simulink model "inv_pen_IC_compare_mar2016"  (R2015b)
settings: Solver=ode45  StartTime=0.0  StopTime=16  MaxStep=0.001  RelTol=1e-3
values from neighbouring files (symbols this model uses):
  g = 9.81    [inverted_pendulum_Feb28_2016.m]
  K1 = K(1)    [inverted_pendulum_Feb28_2016.m]
  K2 = K(2)    [inverted_pendulum_Feb28_2016.m]
  K3 = K(3)    [inverted_pendulum_Feb28_2016.m]
  K4 = K(4)    [inverted_pendulum_Feb28_2016.m]
  l = 0.5    [inverted_pendulum_Feb28_2016.m]
  M = 2    [inverted_pendulum_Feb28_2016.m]
  m = .1    (= 0.1)    [inverted_pendulum_Feb28_2016.m]
libraries: simulink x1
settings Model: Creator=Thomas Chmielewski  LastModifiedBy=DR_C
settings DataIOCC: SaveFormat=Array  SignalLoggingSaveFormat=ModelDataLogs
settings OptimizationCC: ExpressionDepthLimit=2147483647  InitFltsAndDblsToZero=on
settings DebuggingCC: SaveWithParameterizedLinksMsg=none  UnderspecifiedInitializationDetection=Classic  MergeDetectMultiDrivingBlocksExec=none  SolverPrmCheckMsg=warning  FcnCallInpInsideContextMsg=UseLocalSettings  StateNameClashWarn=warning
settings HardwareCC: ProdBitPerPointer=32  ProdLargestAtomicFloat=None  ProdIntDivRoundTo=Undefined  ProdEndianess=Unspecified  ProdWordSize=32  ProdHWDeviceType=32-bit Generic
settings GRTTargetCC: TargetFcnLib=ansi_tfl_tmw.mat  GeneratePreprocessorConditionals=Disable all  CombineOutputUpdateFcns=off  GRTInterface=on
settings ConfigComp: CovModelRefEnable=Off  CovSFcnEnable=off

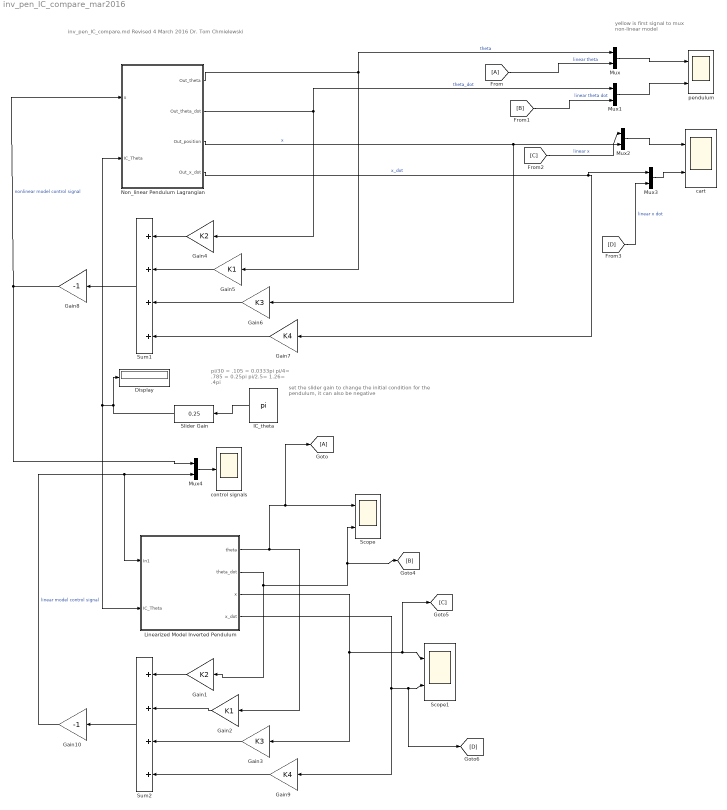
== system inv_pen_IC_compare_mar2016 ==
  note: set the slider gain to change the initial condition
      | for the pendulum, it can also be negative
  note: inv_pen_IC_compare.md
      | Revised 4 March 2016
      | Dr. Tom Chmielewski
  note: yellow is first signal to mux
      | non-linear model
  note: pi/30 = .105 = 0.0333pi
      | pi/4= .785 = 0.25pi
      | pi/2.5= 1.26= .4pi
  " cart" : Scope  NumInputPorts=2
  " control signals" : Scope
  " pendulum" : Scope  NumInputPorts=2
  Display : Display
  Gain1 : Gain  Gain=K2
  Gain10 : Gain  Gain=-1
  Gain2 : Gain  Gain=K1
  Gain3 : Gain  Gain=K3
  Gain4 : Gain  Gain=K2
  Gain5 : Gain  Gain=K1
  Gain6 : Gain  Gain=K3
  Gain7 : Gain  Gain=K4
  Gain8 : Gain  Gain=-1
  Gain9 : Gain  Gain=K4
  IC_theta : Constant  Value=pi
  Linearized Model Inverted Pendulum : Subsystem
  Mux{,1..4} (5 alike) : Mux  Inputs=2
  Non_linear Pendulum Lagrangian : Subsystem
  Scope : Scope  NumInputPorts=2
  Scope1 : Scope  NumInputPorts=2
  Slider Gain : simulink/Math Operations/Slider Gain  low=-0.4  gain=0.25  high=0.4
  Sum1 : Sum  Inputs=++++
  Sum2 : Sum  Inputs=++++
  wires:
  Gain4/1 -> Sum1/1
  Gain5/1 -> Sum1/2
  Gain6/1 -> Sum1/3
  Gain7/1 -> Sum1/4
  Sum1/1 -> Gain8/1
  Non_linear Pendulum Lagrangian/3(Out_position) -> Gain6/1, Mux2/1  "x"
  Gain8/1 -> Mux4/1, Non_linear Pendulum Lagrangian/1(u)  "nonlinear model control signal"
  Non_linear Pendulum Lagrangian/4(Out_x_dot) -> Gain7/1, Mux3/1  "x_dot"
  Non_linear Pendulum Lagrangian/1(Out_theta) -> Mux/1, Gain5/1  "theta"
  Non_linear Pendulum Lagrangian/2(Out_theta_dot) -> Gain4/1, Mux1/1  "theta_dot"
  Gain1/1 -> Sum2/1
  Gain2/1 -> Sum2/2
  Gain3/1 -> Sum2/3
  Gain9/1 -> Sum2/4
  Sum2/1 -> Gain10/1
  Linearized Model Inverted Pendulum/1(theta) -> Gain2/1, Scope/1, [A]
  Linearized Model Inverted Pendulum/2(theta_dot) -> Gain1/1, Scope/2, [B]
  Linearized Model Inverted Pendulum/3(x) -> Gain3/1, Scope1/1, [C]
  Linearized Model Inverted Pendulum/4(x_dot) -> Gain9/1, Scope1/2, [D]
  Mux/1 -> " pendulum"/1
  Mux1/1 -> " pendulum"/2
  Mux2/1 -> " cart"/1
  Mux3/1 -> " cart"/2
  [B] -> Mux1/2  "linear theta dot"
  [C] -> Mux2/2  "linear x"
  [D] -> Mux3/2  "linear x dot"
  [A] -> Mux/2  "linear theta"
  Gain10/1 -> Linearized Model Inverted Pendulum/1(In1), Mux4/2  "linear model control signal"
  Slider Gain/1 -> Non_linear Pendulum Lagrangian/2(IC_Theta), Linearized Model Inverted Pendulum/2(IC_Theta), Display/1
  IC_theta/1 -> Slider Gain/1
  Mux4/1 -> " control signals"/1

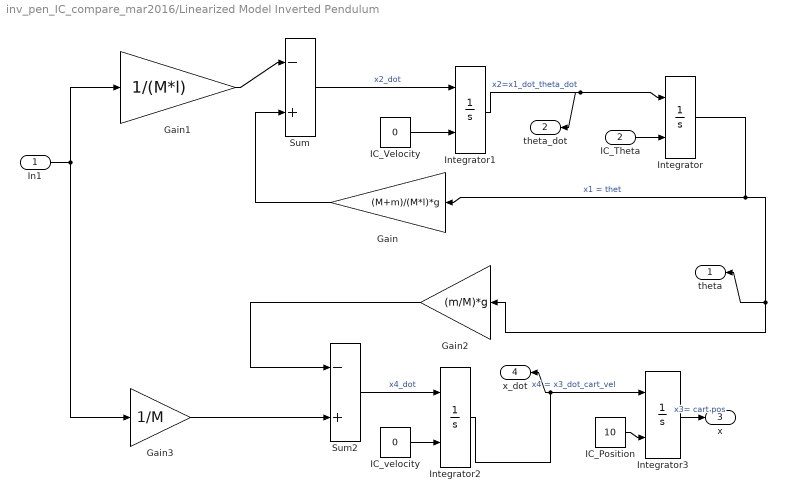
== system inv_pen_IC_compare_mar2016/Linearized Model Inverted Pendulum ==
  In1 : Inport
  IC_Theta : Inport  Port=2
  Gain : Gain  Gain=(M+m)/(M*l)*g
  Gain1 : Gain  Gain=1/(M*l)
  Gain2 : Gain  Gain=(m/M)*g
  Gain3 : Gain  Gain=1/M
  IC_Position : Constant  Value=10
  IC_Velocity : Constant  Value=0
  IC_velocity : Constant  Value=0
  Integrator{,1..3} (4 alike) : Integrator  InitialConditionSource=external
  Sum : Sum  Inputs=|-+
  Sum2 : Sum  Inputs=-+
  theta : Outport
  theta_dot : Outport  Port=2
  x : Outport  Port=3
  x_dot : Outport  Port=4
  wires:
  Integrator/1 -> Gain/1, Gain2/1, theta/1  "x1 = thet"
  Integrator1/1 -> Integrator/1, theta_dot/1  "x2=x1_dot_theta_dot"
  Sum/1 -> Integrator1/1  "x2_dot"
  Gain/1 -> Sum/2
  Gain1/1 -> Sum/1
  Integrator2/1 -> Integrator3/1, x_dot/1  "x4 = x3_dot_cart_vel"
  Sum2/1 -> Integrator2/1  "x4_dot"
  Gain2/1 -> Sum2/1
  Gain3/1 -> Sum2/2
  IC_Theta/1 -> Integrator/2
  In1/1 -> Gain3/1, Gain1/1
  IC_velocity/1 -> Integrator2/2
  IC_Position/1 -> Integrator3/2
  IC_Velocity/1 -> Integrator1/2
  Integrator3/1 -> x/1  "x3= cart pos"

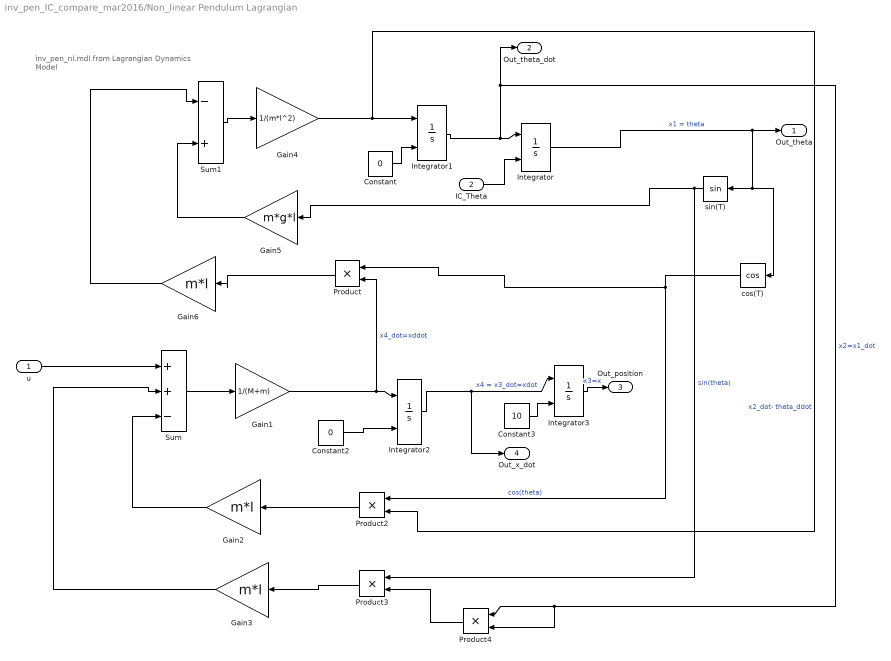
== system inv_pen_IC_compare_mar2016/Non_linear Pendulum Lagrangian ==
  note: inv_pen_nl.mdl
      | from Lagrangian Dynamics Model
  u : Inport
  IC_Theta : Inport  Port=2
  Constant : Constant  Value=0
  Constant2 : Constant  Value=0
  Constant3 : Constant  Value=10
  Gain1 : Gain  Gain=1/(M+m)
  Gain2 : Gain  Gain=m*l
  Gain3 : Gain  Gain=m*l
  Gain4 : Gain  Gain=1/(m*l^2)
  Gain5 : Gain  Gain=m*g*l
  Gain6 : Gain  Gain=m*l
  Integrator{,1..3} (4 alike) : Integrator  InitialConditionSource=external
  Product{,2..4} (4 alike) : Product  RndMeth=Zero
  Sum : Sum  Inputs=++-
  Sum1 : Sum  Inputs=-+
  cos(T) : Trigonometry  Operator=cos
  sin(T) : Trigonometry
  Out_theta : Outport
  Out_theta_dot : Outport  Port=2
  Out_position : Outport  Port=3
  Out_x_dot : Outport  Port=4
  wires:
  Integrator1/1 -> Integrator/1, Out_theta_dot/1, Product4/1, Product4/2  "x2=x1_dot"
  Gain4/1 -> Integrator1/1, Product2/2  "x2_dot- theta_ddot"
  Integrator2/1 -> Integrator3/1, Out_x_dot/1  "x4 = x3_dot=xdot"
  Gain1/1 -> Integrator2/1, Product/2  "x4_dot=xddot"
  Integrator/1 -> Out_theta/1, sin(T)/1, cos(T)/1  "x1 = theta"
  Integrator3/1 -> Out_position/1  "x3=x"
  Sum/1 -> Gain1/1
  sin(T)/1 -> Gain5/1, Product3/1  "sin(theta)"
  Sum1/1 -> Gain4/1
  cos(T)/1 -> Product2/1, Product/1  "cos(theta)"
  Constant/1 -> Integrator1/2
  IC_Theta/1 -> Integrator/2
  Constant2/1 -> Integrator2/2
  Constant3/1 -> Integrator3/2
  u/1 -> Sum/1
  Gain2/1 -> Sum/3
  Product2/1 -> Gain2/1
  Gain3/1 -> Sum/2
  Product3/1 -> Gain3/1
  Product4/1 -> Product3/2
  Gain5/1 -> Sum1/2
  Gain6/1 -> Sum1/1
  Product/1 -> Gain6/1
